simulink model "switch_temp"  (Simulink 7.8)
settings: Solver=ode45  StartTime=0.0  StopTime=10.0  RelTol=1e-3
values from neighbouring files (symbols this model uses):
  A1 = [0 1 ; -1 -2]    [switch_test1.m]
undefined symbols (not defined in the file or in its folder): A2, B1, B2, C1, C2, D1, D2, theta0
libraries: simulink x1
settings Model: Creator=rpichard  LastModifiedBy=rpichard

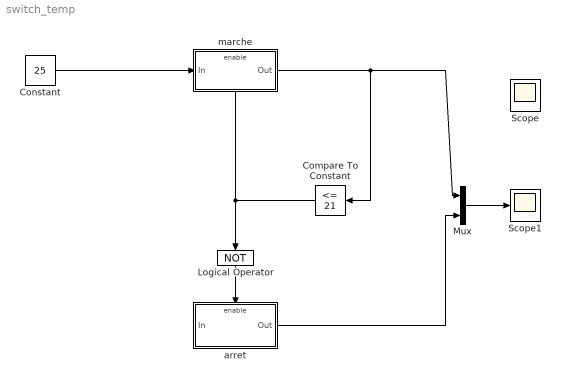
== system switch_temp ==
  Compare To Constant : simulink/Logic and Bit Operations/Compare To Constant  relop=<=  const=21  OutDataTypeStr=boolean
  Constant : Constant  Value=25
  Logical Operator : Logic  Operator=NOT  Inputs=1
  Mux : Mux  Inputs=2
  Scope : Scope
  Scope1 : Scope
  arret : Subsystem  TreatAsAtomicUnit=on
  marche : Subsystem  TreatAsAtomicUnit=on
  wires:
  Constant/1 -> marche/1(In)
  marche/1(Out) -> Compare To Constant/1, Mux/1
  Compare To Constant/1 -> marche/Enable, Logical Operator/1
  Logical Operator/1 -> arret/Enable
  arret/1(Out) -> Mux/2
  Mux/1 -> Scope1/1

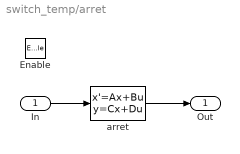
== system switch_temp/arret ==
  In : Inport
  Enable : EnablePort
  arret : StateSpace  A=A2  B=B2  C=C2  D=D2  X0=[21]'
  Out : Outport
  wires:
  arret/1 -> Out/1
  In/1 -> arret/1

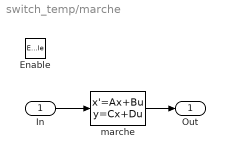
== system switch_temp/marche ==
  In : Inport
  Enable : EnablePort  StatesWhenEnabling=reset
  marche : StateSpace  A=A1  B=B1  C=C1  D=D1  X0=[theta0]'
  Out : Outport  OutputWhenDisabled=reset  InitialOutput=0
  wires:
  In/1 -> marche/1
  marche/1 -> Out/1
